simulink model "controllerlab0"  (Simulink 6.5)
settings: Solver=ode45  SolverMode=SingleTasking  StartTime=0.0  StopTime=total_time  FixedStep=0.001  MaxStep=.001  RelTol=1e-5
values from neighbouring files (symbols this model uses):
  UnitStepVal = 2.0    (= 2)    [LabReport0.m]
settings Model: Creator=abecker5  LastModifiedBy=abecker5  BufferReuse=off
settings DataIOCC: LimitDataPoints=off
settings OptimizationCC: BooleanDataType=off  InlineInvariantSignals=on  OptimizeBlockIOStorage=off  BufferReuse=off  ExpressionFolding=off  LocalBlockOutputs=off
settings DebuggingCC: SolverPrmCheckMsg=none  MultiTaskDSMMsg=warning  MultiTaskCondExecSysMsg=none
settings RTWCC: SystemTargetFile=wincon.tlc  MakeCommand=make_wc  TemplateMakefile=wc_default_tmf  Description=WinCon Target  ProcessScript=wincon_make_rtw_hook  IncludeERTFirstTime=on
settings STFCustomTargetCC: TargetFcnLib=ansi_tfl_tmw.mat  GenFloatMathFcnCalls=ANSI_C  ModelReferenceCompliant=off  SystemTargetFile=wincon.tlc
settings GRTTargetCC: ModelReferenceCompliant=off  MatFileLogging=off  ExtMode=on  ExtModeTransport=2  ExtModeMexFile=wc_comm
settings CustomProperty: Value=on

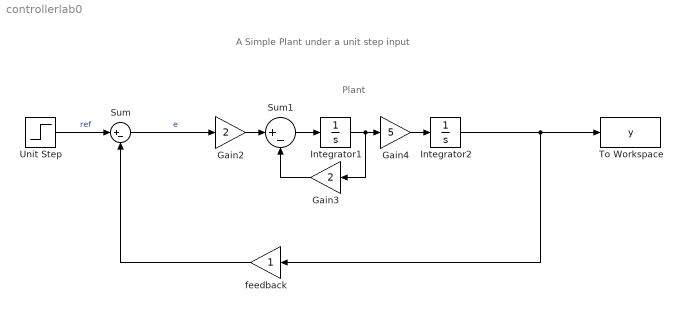
== system controllerlab0 ==
  note: Plant
  note: A Simple Plant under a unit step input
  Gain2 : Gain  Gain=2
  Gain3 : Gain  Orientation=left  Gain=2
  Gain4 : Gain  Gain=5
  Integrator1 : Integrator
  Integrator2 : Integrator
  Sum : Sum  Inputs=|+-
  Sum1 : Sum  Inputs=|+-
  To Workspace : ToWorkspace  VariableName=y  SampleTime=-1  SaveFormat=Array
  Unit Step : Step  Time=0  After=UnitStepVal  SampleTime=0
  feedback : Gain  Orientation=left
  wires:
  Sum1/1 -> Integrator1/1
  Gain4/1 -> Integrator2/1
  Integrator2/1 -> To Workspace/1, feedback/1
  feedback/1 -> Sum/2
  Gain2/1 -> Sum1/1
  Unit Step/1 -> Sum/1  "ref"
  Integrator1/1 -> Gain4/1, Gain3/1
  Sum/1 -> Gain2/1  "e"
  Gain3/1 -> Sum1/2
